simulink model "hmiTestv0"  (R2017a)
settings: Solver=FixedStepAuto  StartTime=0.0  StopTime=inf  RelTol=1e-3
undefined symbols (not defined in the file): vrrotmat2vec
libraries: vrlib x3, myo_lib x3, dspstat3 x2, aerolibconvert2 x1, sldrtlib x1
settings Model: Creator=ricardog  LastModifiedBy=ricardog
settings SolverCC: AutoInsertRateTranBlk=on

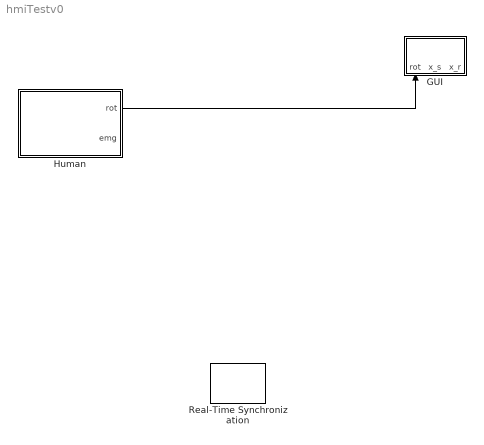
== system hmiTestv0 ==
  GUI : Subsystem
  Human : Subsystem
  Real-Time Synchronization : sldrtlib/Real-Time Synchronization  SampleTime=0.01  MaxMissedTicks=50  ShowMissedTicks=off  YieldWhenWaiting=off
  wires:
  Human/1(rot) -> GUI/1(rot)

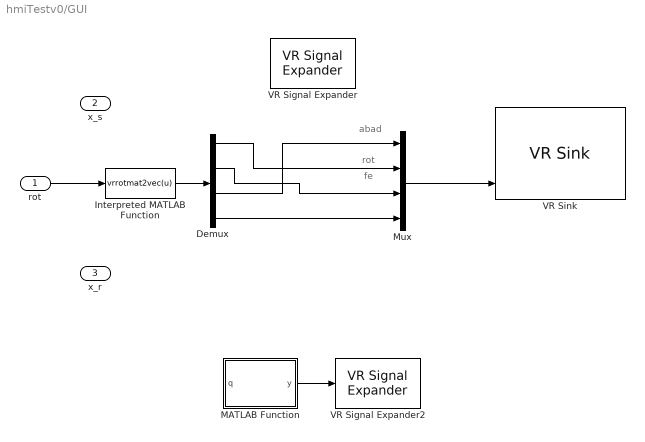
== system hmiTestv0/GUI ==
  note: fe
  note: rot
  note: abad
  rot : Inport
  x_s : Inport  Port=2
  x_r : Inport  Port=3
  Demux : Demux
  Interpreted MATLAB Function : MATLABFcn  MATLABFcn=vrrotmat2vec(u)
  MATLAB Function : MATLAB Function  TreatAsAtomicUnit=on
  Mux : Mux
  VR Signal Expander : vrlib/VR Signal Expander  outwidth=4  outidx=[4]
      settings: SourceProductName=Simulink 3D Animation  SourceProductBaseCode=VR
  VR Signal Expander2 : vrlib/VR Signal Expander  outwidth=3  outidx=[1 2]
      settings: SourceProductName=Simulink 3D Animation  SourceProductBaseCode=VR
  VR Sink : vrlib/VR Sink  InstantiateOnLoad=on  SampleTime=0.1  ViewEnable=on  RemoteChange=off  RemoteView=off  FieldsWritten=Forearm.rotation.4.1.1.double#Forearm.translation.3.1.1.double#UpperArm.rotation.4.1.1.double  WorldFileName=C:\Users\ricardog\Documents\Workspace\IterativeSynergyLearning\GUI\VR\armTargetsVR.wrl  AutoView=on  VideoDimensions=[]  AllowVariableSize=off  FigureProperties="{'Position', 'Name', 'Viewpoint', 'CameraBound', 'CameraDirection', 'CameraPosition', 'CameraUpVector', 'ZoomFactor', 'Antialiasing', 'Headlight', 'Lighting', 'NavPanel', 'Sound', 'StatusBar', 'Stereo3D', 'Stereo3DCameraOffset', 'Stereo3DHIT', 'ToolBar', 'Textures', 'Transparency', 'Triad', 'Wireframe', 'NavZones', 'NavMode', 'NavSpeed', 'CaptureFileFormat', 'CaptureFileName', 'Record2DCompressMethod', 'Record2DCompressQuality', 'Record2D', 'Record2DFileName', 'Record2DFPS'; [5.0000000000000000e+00   9.2000000000000000e+01   5.7600000000000000e+02   3.5000000000000000e+02], '', 'Side view', 'on', [0.0000000000000000e+00   0.0000000000000000e+00  -1.0000000000000000e+00], [0.0000000000000000e+00   0.0000000000000000e+00   0.0000000000000000e+00], [0.0000000000000000e+00   1.0000000000000000e+00   0.0000000000000000e+00], [1.0000000000000000e+00], 'on', 'on', 'on', 'halfbar', 'on', 'on', 'off', [1.0000000149011612e-01], [0.0000000000000000e+00], 'on', 'on', 'on', 'none', 'off', 'off', 'fly', 'normal', 'tif', '%f_anim_%n.tif', 'auto', [7.5000000000000000e+01], 'off', '%f_anim_%n.avi', 'auto'}"
      settings: SourceProductBaseCode=VR
  wires:
  MATLAB Function/1(y) -> VR Signal Expander2/1
  Interpreted MATLAB Function/1 -> Demux/1
  Demux/4 -> Mux/4
  Mux/1 -> VR Sink/3
  Demux/1 -> Mux/2
  Demux/3 -> Mux/1
  rot/1 -> Interpreted MATLAB Function/1
  Demux/2 -> Mux/3

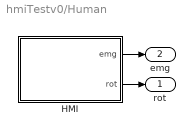
== system hmiTestv0/Human ==
  HMI : Subsystem
  rot : Outport
  emg : Outport  Port=2
  wires:
  HMI/1(emg) -> emg/1
  HMI/2(rot) -> rot/1

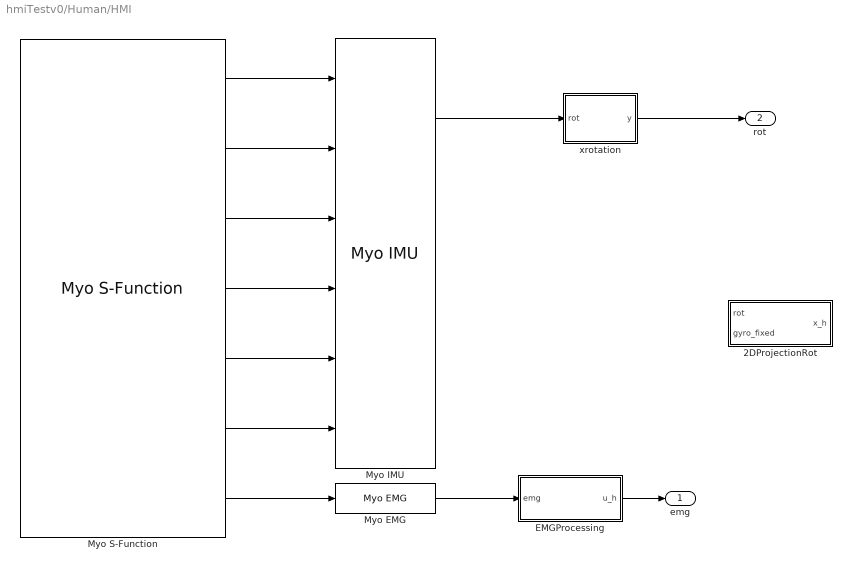
== system hmiTestv0/Human/HMI ==
  2DProjectionRot : Subsystem
  EMGProcessing : Subsystem
  Myo EMG : myo_lib/Myo EMG
  Myo IMU : myo_lib/Myo IMU
  Myo S-Function : myo_lib/Myo S-Function  emgEnabled=1  countMyos=1
  xrotation : MATLAB Function  TreatAsAtomicUnit=on
  emg : Outport
  rot : Outport  Port=2
  wires:
  Myo S-Function/3 -> Myo IMU/3
  Myo S-Function/7 -> Myo EMG/1
  Myo S-Function/4 -> Myo IMU/4
  Myo S-Function/5 -> Myo IMU/5
  Myo S-Function/2 -> Myo IMU/2
  Myo S-Function/1 -> Myo IMU/1
  Myo S-Function/6 -> Myo IMU/6
  Myo EMG/1 -> EMGProcessing/1(emg)
  EMGProcessing/1(u_h) -> emg/1
  Myo IMU/2 -> xrotation/1(rot)
  xrotation/1(y) -> rot/1

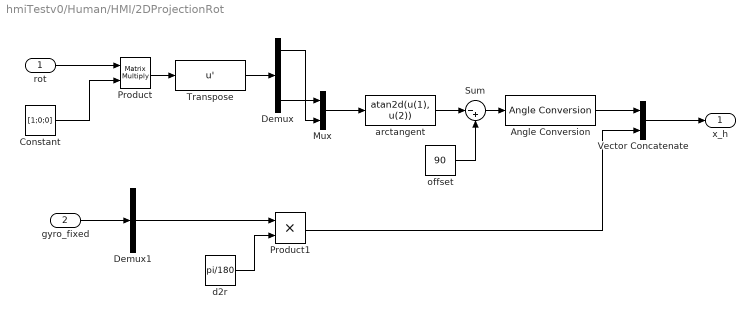
== system hmiTestv0/Human/HMI/2DProjectionRot ==
  rot : Inport
  gyro_fixed : Inport  Port=2
  Angle Conversion : aerolibconvert2/Angle Conversion  IU=deg  OU=rad
  Constant : Constant  Value=[1;0;0]  VectorParams1D=off
  Demux : Demux  Outputs=3
  Demux1 : Demux  Outputs=3
  Mux : Mux  Inputs=2
  Product : Product  Multiplication=Matrix(*)
  Product1 : Product
  Sum : Sum  Inputs=|-+
  Transpose : MATLABFcn  MATLABFcn=u'  Output1D=off
  Vector Concatenate : Concatenate
  arctangent : MATLABFcn  MATLABFcn=atan2d(u(1), u(2))
  d2r : Constant  Value=pi/180
  offset : Constant  Value=90
  x_h : Outport
  wires:
  rot/1 -> Product/1
  Product/1 -> Transpose/1
  Constant/1 -> Product/2
  Transpose/1 -> Demux/1
  Mux/1 -> arctangent/1
  Demux/1 -> Mux/2
  Demux/3 -> Mux/1
  Vector Concatenate/1 -> x_h/1
  gyro_fixed/1 -> Demux1/1
  arctangent/1 -> Sum/1
  offset/1 -> Sum/2
  Sum/1 -> Angle Conversion/1
  Angle Conversion/1 -> Vector Concatenate/1
  Demux1/2 -> Product1/1
  d2r/1 -> Product1/2
  Product1/1 -> Vector Concatenate/2

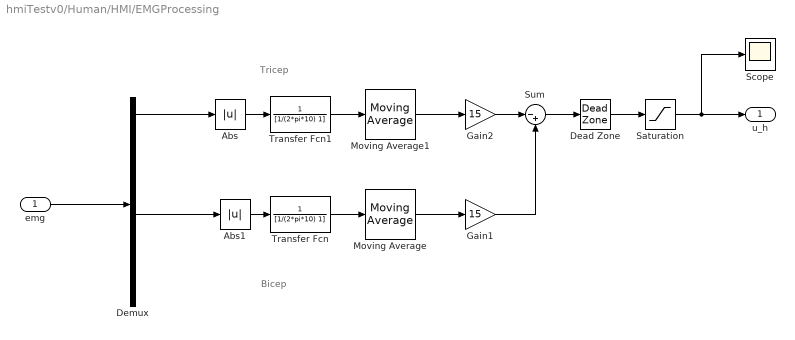
== system hmiTestv0/Human/HMI/EMGProcessing ==
  note: Tricep
  note: Bicep
  emg : Inport
  Abs : Abs
  Abs1 : Abs
  Dead Zone : DeadZone  SaturateOnIntegerOverflow=on
  Demux : Demux  Outputs=8
  Gain1 : Gain  Gain=15
  Gain2 : Gain  Gain=15
  Moving Average : dspstat3/Moving Average  Method=Sliding window  SpecifyWindowLength=on  WindowLength=1000  ForgettingFactor=0.9  SimulateUsing=Code generation
  Moving Average1 : dspstat3/Moving Average  Method=Sliding window  SpecifyWindowLength=on  WindowLength=1000  ForgettingFactor=0.9  SimulateUsing=Code generation
  Saturation : Saturate  UpperLimit=3  LowerLimit=-3
  Scope : Scope
  Sum : Sum  Inputs=|-+
  Transfer Fcn : TransferFcn  Denominator=[1/(2*pi*10) 1]
  Transfer Fcn1 : TransferFcn  Denominator=[1/(2*pi*10) 1]
  u_h : Outport
  wires:
  Transfer Fcn/1 -> Moving Average/1
  Moving Average/1 -> Gain1/1
  Moving Average1/1 -> Gain2/1
  Demux/5 -> Abs1/1
  Demux/1 -> Abs/1
  Abs1/1 -> Transfer Fcn/1
  Transfer Fcn1/1 -> Moving Average1/1
  Abs/1 -> Transfer Fcn1/1
  emg/1 -> Demux/1
  Gain1/1 -> Sum/2
  Gain2/1 -> Sum/1
  Saturation/1 -> Scope/1, u_h/1
  Sum/1 -> Dead Zone/1
  Dead Zone/1 -> Saturation/1

== matlab function hmiTestv0/Human/HMI/xrotation ==
  data: rot input; y output
function y = fcn(rot)

y = roty(90)*rot;

== matlab function hmiTestv0/GUI/MATLAB Function ==
  data: q input; y output
function y = fcn(q)
% Shoulder location offset transformation
% mT01 = T(0,0,0,-pi/2);
% mT02 = T(pi/2,0,0,-pi/2);
% % Shoulder abduction/adduction
% mT1 = T(0,0,0,q(1));
% % Shoulder flexion/extension
% mT2 = T(-pi/2,0,0,q(2)-pi/2);
% % Shoulder rotation
% mT3 = T(-pi/2,0,la,q(3));
y=0
